simulink model "ANNmreza"  (R2013a)
settings: Solver=ode45  StartTime=0.0  StopTime=10.0  RelTol=1e-3
values from neighbouring files (symbols this model uses):
  fazebolesti = str2double(get(hObject,'string'))    [GUIANNmodel.m]
  fizickisimptomi = str2double(get(hObject,'string'))    [GUIANNmodel.m]
  nacinprijenosa = str2double(get(hObject,'string'))    [GUIANNmodel.m]
  opasnostpozivot = str2double(get(hObject,'string'))    [GUIANNmodel.m]
  testiranje = str2double(get(hObject,'string'))    [GUIANNmodel.m]
libraries: neural x106
(part 3 of 3)

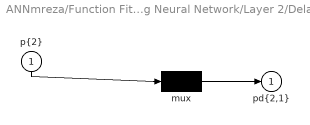
== system ANNmreza/Function Fitting Neural Network/Layer 2/Delays 1 ==
  "p{2}" : Inport  PortDimensions=100
      mask Display: e = 0.06;c1 = [120 230 180]/255;c2 = ([120 230 180]+0)/(256+128);c3 = ([120 230 180]+128)/(256+128);patch([0 1 1 0],[0 0 1 1],c1);patch([0 1 1 1-e 1-e 0+e],[0 0 1 1-e 0+e 0+e],c2);patch([0 0 1 1-e 0+e 0+e],[0 1 1 1-e 1-e 0+e],c3);plot([0 1 1 0 0],[0 0 1 1 0]);
  mux : Mux  Inputs=1
      mask Display: e = 0.06;c1 = [120 150 230]/255;c2 = ([120 150 230]+0)/383;c3 = ([120 150 230]+128)/383;patch([0 1 1 0],[0 0 1 1],c1);patch([0 1 1 1-e 1-e 0+e],[0 0 1 1-e 0+e 0+e],c2);patch([0 0 1 1-e 0+e 0+e],[0 1 1 1-e 1-e 0+e],c3);plot([0 1 1 0 0],[0 0 1 1 0]);disp('Mux')
  "pd{2,1}" : Outport
      mask Display: e = 0.06;c1 = [120 230 180]/255;c2 = ([120 230 180]+0)/(256+128);c3 = ([120 230 180]+128)/(256+128);patch([0 1 1 0],[0 0 1 1],c1);patch([0 1 1 1-e 1-e 0+e],[0 0 1 1-e 0+e 0+e],c2);patch([0 0 1 1-e 0+e 0+e],[0 1 1 1-e 1-e 0+e],c3);plot([0 1 1 0 0],[0 0 1 1 0]);
  wires:
  "p{2}"/1 -> mux/1
  mux/1 -> "pd{2,1}"/1

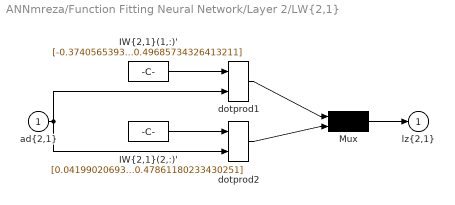
== system ANNmreza/Function Fitting Neural Network/Layer 2/LW{2,1} ==
  "ad{2,1}" : Inport  PortDimensions=100
      mask Display: e = 0.06;c1 = [120 230 180]/255;c2 = ([120 230 180]+0)/(256+128);c3 = ([120 230 180]+128)/(256+128);patch([0 1 1 0],[0 0 1 1],c1);patch([0 1 1 1-e 1-e 0+e],[0 0 1 1-e 0+e 0+e],c2);patch([0 0 1 1-e 0+e 0+e],[0 1 1 1-e 1-e 0+e],c3);plot([0 1 1 0 0],[0 0 1 1 0]);
  "IW{2,1}(1,:)'" : Constant  Value=[-0.3740565393554397;-0.73100880315674588;0.65726221403678231;-0.36297892134445581;0.47801436356631999;0.45369464893779177;-0.26576080951795344;2.5001994183380822;0.41669738859797101;-0.15767275267638381;-1.8037238157035644;-0.35496881358490423;-0.95042495872758359;1.2616280367566799;3.7212207868182716;0.035386526934971997;-0.24165129895746135;-0.51839669464964666;0.8191147490029016;0.3640918801703521;-0.68904089903004428;-1.7577747224324343;-0.058004092763476067;0.48664147187792489;-0.26196833357227534;-0.77727805035526387;0.64715785120187275;1.1393985792375345;0.56670175758625263;-3.2574102403832788;0.27866024911574677;1.1143122293723715;0.59227709143348417;-2.3386963025350096;1.0326184792967017;1.3526843468894088;0.64647771032706403;-0.24823329979867792;4.8633595684581321;0.38178539690057961;1.0460023637149327;0.25286067052248484;0.58445659670157168;2.6741016692716246;-0.85357002290825101;-0.98792720368774367;-1.5082663931015441;1.2069514540226083;-0.53524444353552014;0.6267428855551701;-1.3261374991572474;0.28780586783901696;-0.97381414675325317;0.17955059953320524;0.045320224636750853;-0.14519035584609111;0.19203681610374268;2.0898193299258647;0.089357025270294765;-1.6026709473190266;-1.1174456637944326;-0.78834713348845264;0.20784187304036503;-0.021406091548694148;-0.40843806809621946;0.081063654718474779;-0.071554725375358424;0.89771460498894373;-0.59653984492282985;-0.26045693127567665;1.159926378606388;0.64647185737074775;-0.48794483611388434;-0.044190926484567919;-1.0423052973881339;-0.078323098498364108;0.49423001886643986;0.3076176310866669;4.3063002111586259;-0.89374405439821758;-0.53594378153526778;-0.30739505528266692;-0.27179805373348515;-0.12281864546071704;-0.8137698587541079;-0.083893187766497207;-0.203194725113963;0.68650603099623886;-0.29963432550939706;0.53185880784414885;0.53874691116883433;-0.41048943077934896;-0.30893204495097071;-0.86639752060446495;0.70759629132472468;-0.13613503548851549;0.1268506930729508;0.1908022763606487;0.5796123262178472;0.49685734326413211]
      mask Display: e = 0.06;c1 = [120 150 230]/255;c2 = ([120 150 230]+0)/383;c3 = ([120 150 230]+128)/383;patch([0 1 1 0],[0 0 1 1],c1);patch([0 1 1 1-e 1-e 0+e],[0 0 1 1-e 0+e 0+e],c2);patch([0 0 1 1-e 0+e 0+e],[0 1 1 1-e 1-e 0+e],c3);plot([0 1 1 0 0],[0 0 1 1 0]);disp('weights');
  "IW{2,1}(2,:)'" : Constant  Value=[0.041990206938281691;-0.84253744737520331;-0.34690001893106032;0.48745714207523022;0.42683849050742262;0.39399198371213973;0.10937072823511113;-0.036640153812601543;-0.12863973150818572;0.29709629225916595;-0.063357296278474001;-0.70857726280235478;-0.16732796398788211;0.21795321294040282;-0.1448165234526306;0.56871990421007312;0.70917318882683089;0.52062069632257901;-0.35952413090764546;-0.25124643186181211;0.19397989409268507;0.1576610392224311;-0.84728673466143456;-0.60029496477748256;0.2388680174062929;0.65225612878314998;-0.37030099973456421;-0.59887738334624085;-0.25726500901528204;-0.026337094333636294;-0.58006654541611435;-0.3589284108899442;0.18867430371859398;-0.56225388978886792;-0.31197513761347384;-0.1215893023141045;0.38318536298270894;0.36206317600597121;-0.047977468071858258;-0.72000834298297267;0.10455246513363707;0.063203441385647;0.51695720646007215;-0.019270136010290297;0.16434415787331744;0.39599236813016647;0.042181406588609811;-0.13512621102494685;0.095021479998885022;-0.80048559451330936;-0.15354052195367571;0.49730167129019287;0.29666214981901956;-0.19949215228662559;0.73092547092529647;-0.35068238931875356;-0.10203912687849773;-0.0084154510839019609;0.089386516170709182;-0.52577452051542195;0.27517505301965695;-0.35733595444685673;-0.39825833879308409;0.79152004769656792;0.16118212108057275;-0.40413756907685155;-0.34236082599725415;0.20420686831677673;0.37690864751224812;0.30272007858062278;-0.027860179559109154;0.078208919864318813;-0.51909740968546292;0.28771208087871042;0.081129654266725248;-0.70670187158191733;0.76529567057938641;-0.32153891210256708;-0.037014890132330586;-0.34060494825136939;-0.010421836099145975;0.21856851548708434;-0.16953621225292712;-0.51732332611113296;0.24010787530335997;0.23768949269140285;-0.12876890986413661;0.0033473324633497138;-1.1395528800384709;-0.82302690340317974;-0.61005890222714831;0.78401508043859192;-0.20054142334255282;-0.026467016260054585;-0.54215469804983651;-0.23213468253051314;-0.0048026704245757714;-0.30786134101490004;0.10990403253257368;0.47861180233430251]
      mask Display: e = 0.06;c1 = [120 150 230]/255;c2 = ([120 150 230]+0)/383;c3 = ([120 150 230]+128)/383;patch([0 1 1 0],[0 0 1 1],c1);patch([0 1 1 1-e 1-e 0+e],[0 0 1 1-e 0+e 0+e],c2);patch([0 0 1 1-e 0+e 0+e],[0 1 1 1-e 1-e 0+e],c3);plot([0 1 1 0 0],[0 0 1 1 0]);disp('weights');
  Mux : Mux  Inputs=2
      mask Display: e = 0.06;c1 = [120 150 230]/255;c2 = ([120 150 230]+0)/383;c3 = ([120 150 230]+128)/383;patch([0 1 1 0],[0 0 1 1],c1);patch([0 1 1 1-e 1-e 0+e],[0 0 1 1-e 0+e 0+e],c2);patch([0 0 1 1-e 0+e 0+e],[0 1 1 1-e 1-e 0+e],c3);plot([0 1 1 0 0],[0 0 1 1 0]);disp('Mux');
  dotprod1 : neural/Weight Functions/dotprod
  dotprod2 : neural/Weight Functions/dotprod
  "lz{2,1}" : Outport
      mask Display: e = 0.06;c1 = [120 230 180]/255;c2 = ([120 230 180]+0)/(256+128);c3 = ([120 230 180]+128)/(256+128);patch([0 1 1 0],[0 0 1 1],c1);patch([0 1 1 1-e 1-e 0+e],[0 0 1 1-e 0+e 0+e],c2);patch([0 0 1 1-e 0+e 0+e],[0 1 1 1-e 1-e 0+e],c3);plot([0 1 1 0 0],[0 0 1 1 0]);
  wires:
  "IW{2,1}(1,:)'"/1 -> dotprod1/1
  "ad{2,1}"/1 -> dotprod1/2, dotprod2/2
  dotprod1/1 -> Mux/1
  "IW{2,1}(2,:)'"/1 -> dotprod2/1
  dotprod2/1 -> Mux/2
  Mux/1 -> "lz{2,1}"/1
